simulink model "LQR"  (R2018b)
settings: Solver=VariableStepAuto  StartTime=0.0  StopTime=20  RelTol=1e-3
settings Model: Creator=Pascal  LastModifiedBy=Pascal

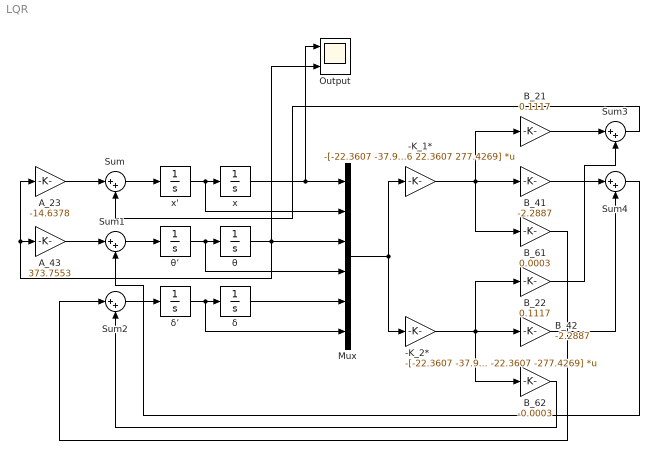
== system LQR ==
  -K_1* : Gain  Gain=-[-22.3607 -37.9597 -197.9191 -26.0606 22.3607 277.4269]  Multiplication=Matrix(K*u)
  -K_2* : Gain  Gain=-[-22.3607 -37.9597 -197.9191 -26.0606 -22.3607 -277.4269]  Multiplication=Matrix(K*u)
  A_23 : Gain  Gain=-14.6378
  A_43 : Gain  Gain=373.7553
  B_21 : Gain  Gain=0.1117
  B_22 : Gain  Gain=0.1117
  B_41 : Gain  Gain=-2.2887
  B_42 : Gain  Gain=-2.2887
  B_61 : Gain  Gain=0.0003
  B_62 : Gain  Gain=-0.0003
  Mux : Mux  Inputs=6
  Output : Scope  NumInputPorts=2
  Sum{,1..4} (5 alike) : Sum  Inputs=|++
  x : Integrator
  x' : Integrator
  δ : Integrator
  δ’ : Integrator
  θ : Integrator  InitialCondition=0.2618
  θ’ : Integrator
  wires:
  x'/1 -> Mux/2, x/1
  -K_2*/1 -> B_22/1, B_42/1, B_62/1
  θ/1 -> A_23/1, A_43/1, Mux/3, Output/2
  Sum4/1 -> Sum1/2
  Sum1/1 -> θ’/1
  B_41/1 -> Sum4/1
  Sum3/1 -> Sum/2
  Sum/1 -> x'/1
  Mux/1 -> -K_2*/1, -K_1*/1
  B_22/1 -> Sum3/2
  Sum2/1 -> δ’/1
  B_62/1 -> Sum2/2
  A_23/1 -> Sum/1
  δ’/1 -> Mux/6, δ/1
  -K_1*/1 -> B_21/1, B_41/1, B_61/1
  B_61/1 -> Sum2/1
  A_43/1 -> Sum1/1
  δ/1 -> Mux/5
  B_21/1 -> Sum3/1
  x/1 -> Output/1, Mux/1
  θ’/1 -> Mux/4, θ/1
  B_42/1 -> Sum4/2
